simulink model "TemporalEvent2"  (R2020b)
settings: Solver=VariableStepAuto  StartTime=0.0  StopTime=10.0  RelTol=1e-3
settings Model: EnablePacing=on  Creator=apple  LastModifiedBy=apple

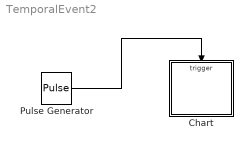
== system TemporalEvent2 ==
  Chart : Stateflow chart  TreatAsAtomicUnit=on
  Pulse Generator : DiscretePulseGenerator  PulseType=Time based  PulseWidth=50
  wires:
  Pulse Generator/1 -> Chart/Trigger

== stateflow chart TemporalEvent2/Chart ==
  state A
    en:fprintf("Entry A");
    du:fprintf("During A");
    ex:fprintf("Exit A");
    state A1
      en:fprintf("Entry A1");
      ex:fprintf("Exit A1");
    (default) -> A1
  state B
    en:fprintf("Entry B");
    du:fprintf("During B");
    ex:fprintf("Exit B");
  (default) -> A
  A -> B : after(3,E)
  (junction 5) -> A1
  A1 -> (junction 5)
  events: E input EITHER_EDGE_EVENT
